simulink model "euler_equation"  (R2024a)
settings: Solver=VariableStepAuto  StartTime=0.0  StopTime=100  RelTol=1e-3
values from neighbouring files (symbols this model uses):
  cbv0 = cb2 * c21 * c1v    [eulerangle (1).m]
  phi0 = 0    [eulerangle (1).m]
  psi0 = 0    [eulerangle (1).m]
  q0 = angle2quat(psi0,theta0,phi0)    [eulerangle (1).m]
  theta0 = 0.0059    [eulerangle (1).m]
libraries: aerolibanim x1, simulink_extras x1

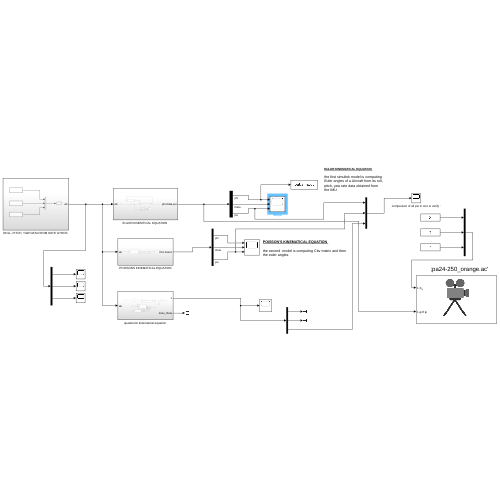
[thumbnail: Simulink's stored preview of the top-level diagram]
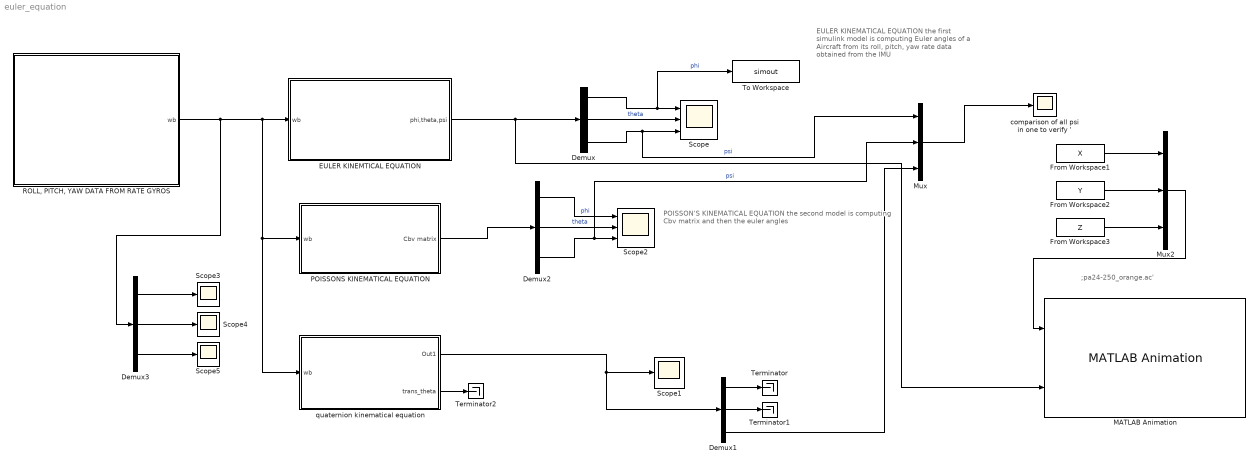
== system euler_equation ==
  note: ;pa24-250_orange.ac'
  note: POISSON'S KINEMATICAL EQUATION
      |
      | the second model is computing Cbv matrix and then the euler angles
  note: EULER KINEMATICAL EQUATION
      |
      | the first simulink model is computing Euler angles of a Aircraft from its roll, pitch, yaw rate data obtained from the IMU
  Demux{,1..3} (4 alike) : Demux  Outputs=3
  "EULER KINEMTICAL EQUATION " : Subsystem
  From Workspace1 : FromWorkspace  VariableName=X
  From Workspace2 : FromWorkspace  VariableName=Y
  From Workspace3 : FromWorkspace  VariableName=Z
  MATLAB Animation : aerolibanim/MATLAB Animation  Tag=Matlab Animation 6 DOF  Vehicles=1  Geometries='pa24-250_orange.ac'  BoundingBoxCoordinates=[-50,50,-50,50,-50,100]  CameraOffset=[-150,-50,0]  CameraViewAngle=2  SampleTime=0.05  FigurePosition=[411,-8,739,509]
  Mux : Mux  Inputs=3
  Mux2 : Mux  Inputs=3
  POISSONS KINEMATICAL EQUATION : Subsystem
  "ROLL, PITCH, YAW DATA FROM RATE GYROS " : Subsystem
  Scope : Scope  NumInputPorts=3
  Scope{1,3..5} (4 alike) : Scope
  Scope2 : Scope  NumInputPorts=3
  Terminator : Terminator
  Terminator1 : Terminator
  Terminator2 : Terminator
  To Workspace : ToWorkspace  VariableName=simout  SaveFormat=Timeseries  SampleTime=-1
  comparison of all psi in one to verify ' : Scope
  "quaternion kinematical equation " : Subsystem
  wires:
  Demux/1 -> To Workspace/1, Scope/1  "phi"
  Demux/2 -> Scope/2  "theta"
  Demux/3 -> Mux/1, Scope/3  "psi"
  Demux2/1 -> Scope2/1  "phi"
  Demux2/2 -> Scope2/2  "theta"
  Demux2/3 -> Mux/2, Scope2/3  "psi"
  "EULER KINEMTICAL EQUATION "/1(phi,theta,psi) -> MATLAB Animation/2, Demux/1
  "ROLL, PITCH, YAW DATA FROM RATE GYROS "/1(wb) -> Demux3/1, "quaternion kinematical equation "/1(wb), POISSONS KINEMATICAL EQUATION/1(wb), "EULER KINEMTICAL EQUATION "/1(wb)
  POISSONS KINEMATICAL EQUATION/1(Cbv matrix) -> Demux2/1
  Demux1/2 -> Terminator1/1
  Demux1/1 -> Terminator/1
  Demux1/3 -> Mux/3
  Mux/1 -> comparison of all psi in one to verify '/1
  "quaternion kinematical equation "/1(Out1) -> Demux1/1, Scope1/1
  From Workspace1/1 -> Mux2/1
  From Workspace2/1 -> Mux2/2
  From Workspace3/1 -> Mux2/3
  Mux2/1 -> MATLAB Animation/1
  "quaternion kinematical equation "/2(trans_theta) -> Terminator2/1
  Demux3/1 -> Scope3/1
  Demux3/2 -> Scope4/1
  Demux3/3 -> Scope5/1

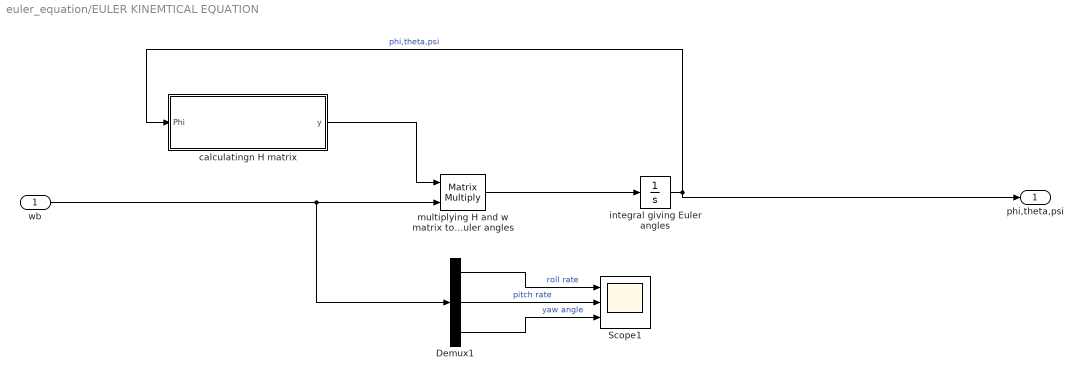
== system euler_equation/EULER KINEMTICAL EQUATION  ==
  wb : Inport
  Demux1 : Demux  Outputs=3
  Scope1 : Scope  NumInputPorts=3
  "calculatingn H matrix " : MATLAB Function  TreatAsAtomicUnit=on
  "integral giving Euler angles " : Integrator  InitialCondition=[phi0 ; theta0 ; psi0]
  "multiplying H and w matrix to rate of change of euler angles " : Product  Multiplication=Matrix(*)
  phi,theta,psi : Outport
  wires:
  wb/1 -> Demux1/1, "multiplying H and w matrix to rate of change of euler angles "/2
  "calculatingn H matrix "/1(y) -> "multiplying H and w matrix to rate of change of euler angles "/1
  "multiplying H and w matrix to rate of change of euler angles "/1 -> "integral giving Euler angles "/1
  Demux1/3 -> Scope1/3  "yaw angle"
  Demux1/1 -> Scope1/1  "roll rate"
  Demux1/2 -> Scope1/2  "pitch rate"
  "integral giving Euler angles "/1 -> phi,theta,psi/1, "calculatingn H matrix "/1(Phi)  "phi,theta,psi"

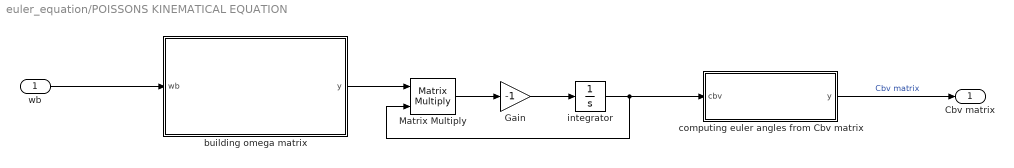
== system euler_equation/POISSONS KINEMATICAL EQUATION ==
  wb : Inport
  " building omega matrix " : MATLAB Function  TreatAsAtomicUnit=on
  Gain : Gain  Gain=-1
  Matrix Multiply : Product  Multiplication=Matrix(*)
  "computing euler angles from Cbv matrix " : MATLAB Function  TreatAsAtomicUnit=on
  "integrator " : Integrator  InitialCondition=cbv0
  Cbv matrix : Outport
  wires:
  Matrix Multiply/1 -> Gain/1
  " building omega matrix "/1(y) -> Matrix Multiply/1
  "computing euler angles from Cbv matrix "/1(y) -> Cbv matrix/1  "Cbv matrix"
  "integrator "/1 -> Matrix Multiply/2, "computing euler angles from Cbv matrix "/1(cbv)
  Gain/1 -> "integrator "/1
  wb/1 -> " building omega matrix "/1(wb)

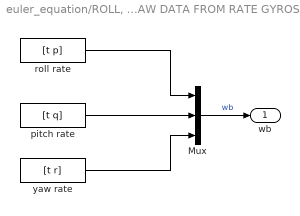
== system euler_equation/ROLL, PITCH, YAW DATA FROM RATE GYROS  ==
  Mux : Mux  Inputs=3
  "pitch rate " : FromWorkspace  VariableName=[t q]
  "roll rate " : FromWorkspace  VariableName=[t p]
  "yaw rate " : FromWorkspace  VariableName=[t r]
  wb : Outport
  wires:
  "pitch rate "/1 -> Mux/2
  "roll rate "/1 -> Mux/1
  "yaw rate "/1 -> Mux/3
  Mux/1 -> wb/1  "wb"

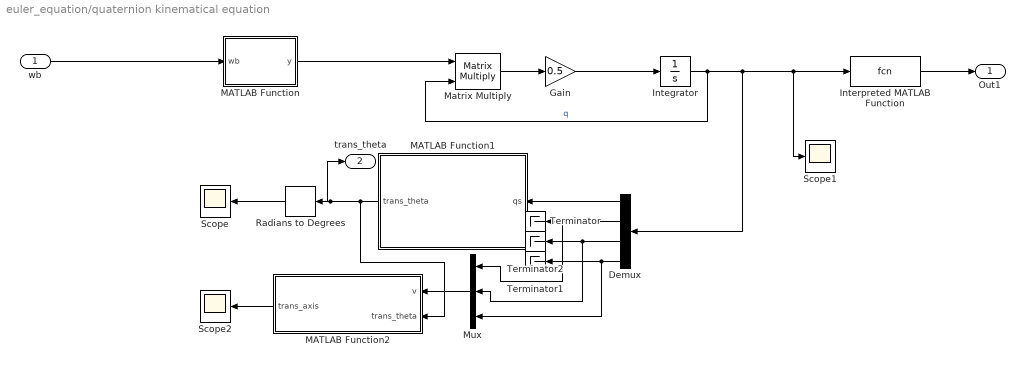
== system euler_equation/quaternion kinematical equation  ==
  wb : Inport
  Demux : Demux
  Gain : Gain  Gain=0.5
  Integrator : Integrator  InitialCondition=q0
  Interpreted MATLAB Function : MATLABFcn  MATLABFcn=fcn
  MATLAB Function : MATLAB Function  TreatAsAtomicUnit=on
  MATLAB Function1 : MATLAB Function  TreatAsAtomicUnit=on
  MATLAB Function2 : MATLAB Function  TreatAsAtomicUnit=on
  Matrix Multiply : Product  Multiplication=Matrix(*)
  Mux : Mux  Inputs=3
  Radians to Degrees : simulink_extras/Transformations/Radians to Degrees
  Scope : Scope
  Scope1 : Scope
  Scope2 : Scope
  Terminator : Terminator
  Terminator1 : Terminator
  Terminator2 : Terminator
  Out1 : Outport
  trans_theta : Outport  Port=2
  wires:
  MATLAB Function/1(y) -> Matrix Multiply/1
  Interpreted MATLAB Function/1 -> Out1/1
  Gain/1 -> Integrator/1
  Integrator/1 -> Demux/1, Scope1/1, Interpreted MATLAB Function/1, Matrix Multiply/2  "q"
  Matrix Multiply/1 -> Gain/1
  wb/1 -> MATLAB Function/1(wb)
  MATLAB Function1/1(trans_theta) -> MATLAB Function2/2(trans_theta), trans_theta/1, Radians to Degrees/1
  Demux/1 -> MATLAB Function1/1(qs)
  Demux/2 -> Mux/1, Terminator/1
  Demux/3 -> Mux/2, Terminator2/1
  Demux/4 -> Terminator1/1, Mux/3
  Mux/1 -> MATLAB Function2/1(v)
  MATLAB Function2/1(trans_axis) -> Scope2/1
  Radians to Degrees/1 -> Scope/1

== matlab function euler_equation/EULER KINEMTICAL EQUATION /calculatingn H matrix  ==
  data: Phi input; y output
function y = euler_kinematical_equation(Phi) 

phi = Phi(1) ; 
theta = Phi(2) ;
psi2 = Phi(3) ;

H = [1 sin(phi)*tan(theta) cos(phi)*tan(theta) ;
    0 cos(phi) -sin(phi) ;
    0 sec(theta)*sin(phi) cos(phi)*sec(theta) ];



y = H;

== matlab function euler_equation/POISSONS KINEMATICAL EQUATION/computing euler angles from Cbv matrix  ==
  data: cbv input; y output
function y = euler_angles_compute(cbv)

c11 = cbv(1,1);
c23 = cbv(2,3);
c33 = cbv(3,3);
c13 = cbv(1,3);
c12 = cbv(1,2);

phi = atan2(c23,c33);
theta = -asin(c13);
psi2 = atan2(c12,c11);

Phi = [phi;theta;psi2];
y = Phi;

== matlab function euler_equation/quaternion kinematical equation /MATLAB Function ==
  data: wb input; y output
function y = fcn(wb)

wx= wb(1) ;
wy= wb(2) ;
wz= wb(3) ;

omega = [
    0 -wx -wy -wz;
    wx 0 wz -wy;
    wy -wz 0 wx;
    wz wy -wx 0];

y = omega;

== matlab function euler_equation/quaternion kinematical equation /MATLAB Function1 ==
  data: qs input; trans_theta output
function trans_theta  = fcn(qs)


trans_theta = 2*acos(complex(qs));

end

== matlab function euler_equation/quaternion kinematical equation /MATLAB Function2 ==
  data: v input; trans_axis output; trans_theta input
function trans_axis = fcn(v,trans_theta)

e = v.*(1/sin(trans_theta/2));


trans_axis = e;

== matlab function euler_equation/POISSONS KINEMATICAL EQUATION/ building omega matrix  ==
  data: wb input; y output
function y = omega_matrix(wb)
p = wb(1) ;
q = wb(2) ;
r = wb(3) ;
omega = [0 -r q ;
    r 0 -p ;
    -q p 0];
y = omega;
